simulink model "sim_AFS"  (R2018a)
settings: Solver=VariableStepAuto  StartTime=0.0  StopTime=10.0  RelTol=1e-3
values from neighbouring files (symbols this model uses):
  a11 = -2*(cf+cr)/m/v    (= -9.36)    [AFS.m]
  a12 = -1-2*(lf*cf-lr*cr)/m/v/v    (= -0.9745984)    [AFS.m]
  a21 = -2*(lf*cf-lr*cr)/iz    (= 12.3270440252)    [AFS.m]
  a22 = -2*(lf*lf*cf+lr*lr*cr)/iz/v    (= -9.16473962264)    [AFS.m]
  b11 = 2*cf/m/v    (= 3.6)    [AFS.m]
  b21 = 2*lf*cf/iz    (= 94.3396226415)    [AFS.m]
  G = input('Without Control (0) or With AFS Control (1) : ')    [AFS.m]
  iz = 159    [AFS.m]
  kgamma = a0/b0    (= 9.48297846524)    [AFS.m]
  n = 18.7    [AFS.m]
  T = 0.0106    [AFS.m]
  tgamma = a0/b0/a1    (= 0.0628247323322)    [AFS.m]
settings Model: Creator=aoki-soya  LastModifiedBy=aoki-soya

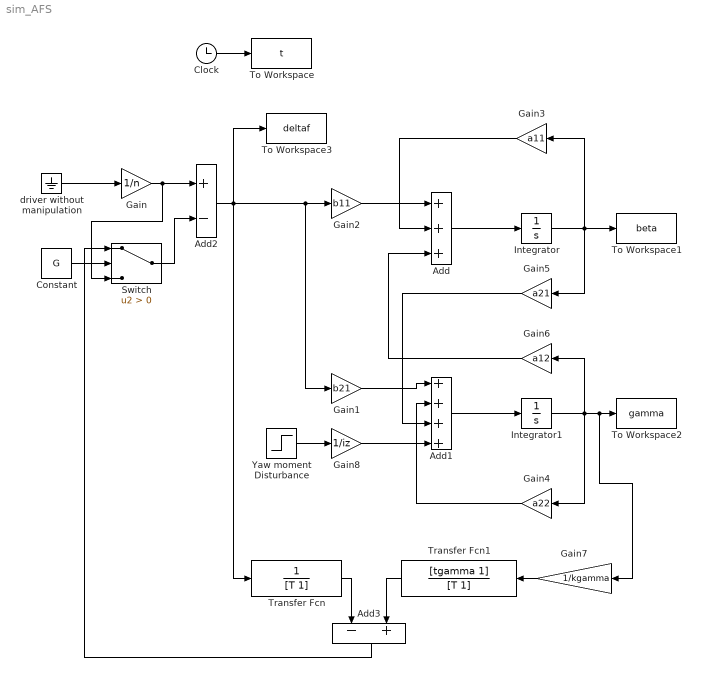
== system sim_AFS ==
  Add : Sum  Inputs=+++
  Add1 : Sum  Inputs=++++
  Add2 : Sum  Inputs=+-
  Add3 : Sum  Inputs=-+
  Clock : Clock
      settings: Decimation=1/mydt
  Constant : Constant  Value=G
  Gain : Gain  Gain=1/n
  Gain1 : Gain  Gain=b21
  Gain2 : Gain  Gain=b11
  Gain3 : Gain  Gain=a11
  Gain4 : Gain  Gain=a22
  Gain5 : Gain  Gain=a21
  Gain6 : Gain  Gain=a12
  Gain7 : Gain  Gain=1/kgamma
  Gain8 : Gain  Gain=1/iz
  Integrator : Integrator
  Integrator1 : Integrator
  Switch : Switch  Criteria=u2 > Threshold
  To Workspace : ToWorkspace  VariableName=t  SaveFormat=Timeseries  SampleTime=-1
  To Workspace1 : ToWorkspace  VariableName=beta  SaveFormat=Timeseries  SampleTime=-1
  To Workspace2 : ToWorkspace  VariableName=gamma  SaveFormat=Timeseries  SampleTime=-1
  To Workspace3 : ToWorkspace  VariableName=deltaf  SaveFormat=Timeseries  SampleTime=-1
  Transfer Fcn : TransferFcn  Denominator=[T 1]
  Transfer Fcn1 : TransferFcn  Numerator=[tgamma 1]  Denominator=[T 1]
  Yaw moment Disturbance : Step  SampleTime=0
  driver without manipulation : Ground
  wires:
  driver without manipulation/1 -> Gain/1
  Gain1/1 -> Add1/1
  Gain5/1 -> Add1/3
  Gain3/1 -> Add/2
  Add1/1 -> Integrator1/1
  Add/1 -> Integrator/1
  Add2/1 -> Transfer Fcn/1, To Workspace3/1, Gain1/1, Gain2/1
  Gain2/1 -> Add/1
  Clock/1 -> To Workspace/1
  Integrator1/1 -> Gain6/1, Gain4/1, Gain7/1, To Workspace2/1
  Integrator/1 -> Gain5/1, Gain3/1, To Workspace1/1
  Gain4/1 -> Add1/2
  Gain6/1 -> Add/3
  Gain/1 -> Switch/3, Add2/1
  Switch/1 -> Add2/2
  Gain7/1 -> Transfer Fcn1/1
  Transfer Fcn/1 -> Add3/1
  Transfer Fcn1/1 -> Add3/2
  Add3/1 -> Switch/1
  Yaw moment Disturbance/1 -> Gain8/1
  Gain8/1 -> Add1/4
  Constant/1 -> Switch/2
